simulink model "MB_Example_01"  (R2018a)
settings: Solver=VariableStepAuto  StartTime=0.0  StopTime=10.0  RelTol=1e-3
settings Model: Creator=Win10  LastModifiedBy=win10

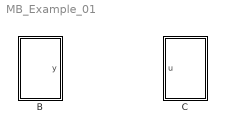
== system MB_Example_01 ==
  B : Subsystem
  C : Subsystem

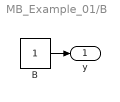
== system MB_Example_01/B ==
  B : Constant
  y : Outport
  wires:
  B/1 -> y/1

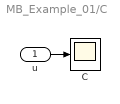
== system MB_Example_01/C ==
  u : Inport
  C : Scope
  wires:
  u/1 -> C/1
